simulink model "New_Energy_Model"  (R2019a)
settings: Solver=VariableStepAuto  StartTime=0.0  StopTime=834  RelTol=1e-3
settings Model: Creator=eabrowning  LastModifiedBy=eabrowning

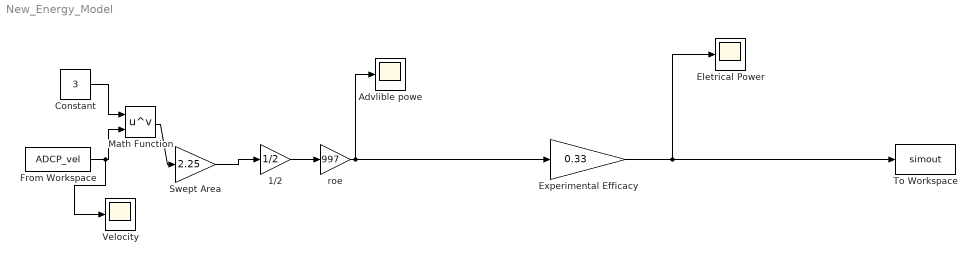
== system New_Energy_Model ==
  1/2 : Gain  Gain=1/2
  "Advlible powe " : Scope
  Constant : Constant  Value=3
  "Eletrical Power " : Scope
  Experimental Efficacy : Gain  Gain=0.33
  From Workspace : FromWorkspace  VariableName=ADCP_vel  OutDataTypeStr=double  OutputAfterFinalValue=Holding final value
  Math Function : Math  Operator=pow  SaturateOnIntegerOverflow=on
  Swept Area : Gain  Gain=2.25
  To Workspace : ToWorkspace  VariableName=simout  SaveFormat=Timeseries  SampleTime=-1
  Velocity : Scope
  roe : Gain  Gain=997
  wires:
  From Workspace/1 -> Velocity/1, Math Function/2
  Swept Area/1 -> 1/2/1
  Math Function/1 -> Swept Area/1
  Constant/1 -> Math Function/1
  roe/1 -> Experimental Efficacy/1, "Advlible powe "/1
  1/2/1 -> roe/1
  Experimental Efficacy/1 -> To Workspace/1, "Eletrical Power "/1
